simulink model "CruiseControl_SLT_6"  (R2017a)
settings: Solver=FixedStepDiscrete  StartTime=0.0  StopTime=2  FixedStep=0.1  RelTol=1e-3  EnableMultiTasking=on
PostLoadFcn:
  | CruiseControl_dd;
undefined symbols (not defined in the file): holdrate, incdec, maxtspeed, mintspeed
settings Model: Creator=The MathWorks Inc.  LastModifiedBy=colosky
settings DataIOCC: LimitDataPoints=on  SaveFormat=Array  SaveOutput=off  SaveTime=off
settings OptimizationCC: DefaultParameterBehavior=Inlined  InlineInvariantSignals=on  ExpressionDepthLimit=2147483647  InitFltsAndDblsToZero=on  NoFixptDivByZeroProtection=on  LifeSpan=inf
settings DebuggingCC: SignalInfNanChecking=warning  SaveWithParameterizedLinksMsg=none  UnderspecifiedInitializationDetection=Classic  MergeDetectMultiDrivingBlocksExec=none  SolverPrmCheckMsg=warning  FcnCallInpInsideContextMsg=warning  UniqueDataStoreMsg=warning  AllowSymbolicDim=off  StateNameClashWarn=warning  StrictBusMsg=ErrorOnBusTreatedAsVector  SFUnexpectedBacktrackingDiag=warning  SFNoUnconditionalDefaultTransitionDiag=warning  SFExecutionAtInitializationDiag=none
settings HardwareCC: ProdBitPerPointer=32  ProdBitPerSizeT=32  ProdBitPerPtrDiffT=32  ProdLargestAtomicFloat=None  ProdIntDivRoundTo=Undefined  ProdEndianess=Unspecified  ProdWordSize=32  ProdHWDeviceType=32-bit Generic
settings ModelReferenceCC: ModelReferenceNumInstancesAllowed=Single  PropagateSignalLabelsOutOfModel=off
settings SFSimCC: SimParseCustomCode=off  MATLABDynamicMemAlloc=off
settings RTWCC: SystemTargetFile=ert.tlc  TemplateMakefile=ert_default_tmf  Description=Embedded Coder  GenerateReport=on  IncludeHyperlinkInReport=on  LaunchReport=on  PortableWordSizes=on  GenerateTraceInfo=on  GenerateTraceReport=on  GenerateTraceReportSl=on  GenerateTraceReportSf=on  GenerateTraceReportEml=on
settings CodeAppCC: IgnoreCustomStorageClasses=off  CustomSymbolStrGlobalVar=$N$M
settings ERTTargetCC: MultiwordLength=2048  GenerateSampleERTMain=on  InlinedParameterPlacement=NonHierarchical  ERTCustomFileTemplate=example_file_process.tlc  ConvertIfToSwitch=off  SuppressUnreachableDefaultCases=off
settings ConfigComp: CovEnable=on  CovScope=ReferencedModels  RecordCoverage=on  CovMetricSettings=dcme  CovModelRefEnable=Off  CovExternalEMLEnable=off  CovSFcnEnable=off  DVMode=DesignErrorDetection  DVMaxProcessTime=3000  DVDisplayUnsatisfiableObjectives=on  DVAutomaticStubbing=off  DVMakeOutputFilesUnique=off  DVModelCoverageObjectives=MCDC  DVMaxTestCaseSteps=500  DVTestSuiteOptimization=CombinedObjectives  DVAssertions=EnableAll  DVProofAssumptions=EnableAll  DVIgnoreCovSatisfied=on  DVCoverageDataFile=CruiseControlCovManual.cvt  DVDetectIntegerOverflow=off  DVDetectDeadLogic=on  DVDetectActiveLogic=on  DVDetectFloatOverflow=off  DVMaxViolationSteps=50  DVSaveExpectedOutput=on  DVHarnessModelFileName=$ModelName$_harness_SLDV  DVReportIncludeGraphics=on  PSAutoStubLUT=off

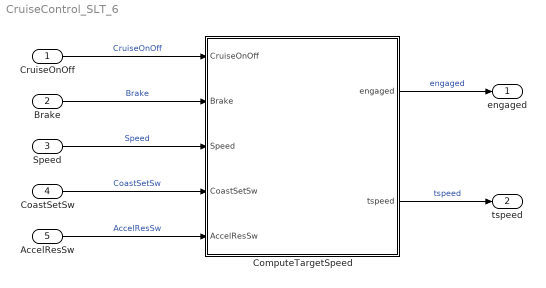
== system CruiseControl_SLT_6 ==
  CruiseOnOff : Inport  PortDimensions=1
  Brake : Inport  Port=2  PortDimensions=1
  Speed : Inport  Port=3  PortDimensions=1
  CoastSetSw : Inport  Port=4  PortDimensions=1
  AccelResSw : Inport  Port=5  PortDimensions=1
  ComputeTargetSpeed : Stateflow chart  TreatAsAtomicUnit=on
  engaged : Outport
  tspeed : Outport  Port=2
  wires:
  AccelResSw/1 -> ComputeTargetSpeed/5(AccelResSw)  "AccelResSw"
  Speed/1 -> ComputeTargetSpeed/3(Speed)  "Speed"
  CoastSetSw/1 -> ComputeTargetSpeed/4(CoastSetSw)  "CoastSetSw"
  CruiseOnOff/1 -> ComputeTargetSpeed/1(CruiseOnOff)  "CruiseOnOff"
  Brake/1 -> ComputeTargetSpeed/2(Brake)  "Brake"
  ComputeTargetSpeed/1(engaged) -> engaged/1  "engaged"
  ComputeTargetSpeed/2(tspeed) -> tspeed/1  "tspeed"

== stateflow chart CruiseControl_SLT_6/ComputeTargetSpeed ==
  state OFF
    en:
    engaged = false;
    tspeed = 0;
  state CRUISE
    state ON
      en:
      engaged = true;
      state Accel
        tspeed = tspeed + incdec;
      state Steady
      state Coast
        tspeed = tspeed - incdec;
      (junction 60) -> Accel
      (junction 57) -> (junction 60) : [after(10*incdec...
          | /holdrate,tick)]
      Accel -> (junction 57) [order 2]
      Steady -> Accel [order 1] : [hasChangedTo(AccelResSw,true) ...
          | && tspeed < maxtspeed]
      Accel -> Steady [order 1] : [!AccelResSw || ...
          | tspeed >= maxtspeed]
      Steady -> (junction 75) [order 3] : [hasChangedTo(CoastSetSw,true)]
      (default) -> (junction 75)
      (junction 75) -> (junction 77) : {tspeed = Speed;}
      (junction 77) -> Steady
      Steady -> Coast [order 2] : [hasChangedTo(CoastSetSw,true) ...
          | && tspeed > mintspeed]
      Coast -> Steady [order 1] : [!CoastSetSw || ...
          | tspeed <= mintspeed]
      (junction 72) -> Coast
      (junction 71) -> (junction 72) : [after(10*incdec...
          | /holdrate,tick)]
      Coast -> (junction 71) [order 2]
    state STANDBY
      en:
      engaged=false;
    (default) -> STANDBY
    ON -> STANDBY : [Brake||Speed> maxtspeed||Speed<mintspeed]
    STANDBY -> (junction 103) : [~Brake && ...
        | Speed<=maxtspeed && ...
        | Speed>=mintspeed]
    (junction 103) -> Steady [order 1] : [hasChangedTo(AccelResSw,true)...
        | &&tspeed!=uint8(0)]
    (junction 103) -> (junction 106) [order 2]
    (junction 106) -> ON : [hasChangedTo(CoastSetSw,true)]
  (default) -> OFF
  OFF -> CRUISE : [CruiseOnOff]
  CRUISE -> OFF : [~CruiseOnOff]
  data: engaged output; CruiseOnOff input; Brake input; Speed input; CoastSetSw input; AccelResSw input; tspeed output; incdec parameter; holdrate parameter; maxtspeed parameter; mintspeed parameter
